simulink library "AttitudeControl"  (R2024a)
settings: Solver=VariableStepAuto  StartTime=0.0  StopTime=10.0  RelTol=1e-3
undefined symbols (not defined in the file): ATC_ANG_PIT_P, ATC_ANG_RLL_P, ATC_ANG_YAW_P, ATC_RAT_PIT_D, ATC_RAT_PIT_I, ATC_RAT_PIT_P, ATC_RAT_RLL_D, ATC_RAT_RLL_I, ATC_RAT_RLL_P, ATC_RAT_YAW_D, ATC_RAT_YAW_I, ATC_RAT_YAW_P
libraries: ArdupilotFunctions x3
settings Model: Creator=igmso  LastModifiedBy=igmso

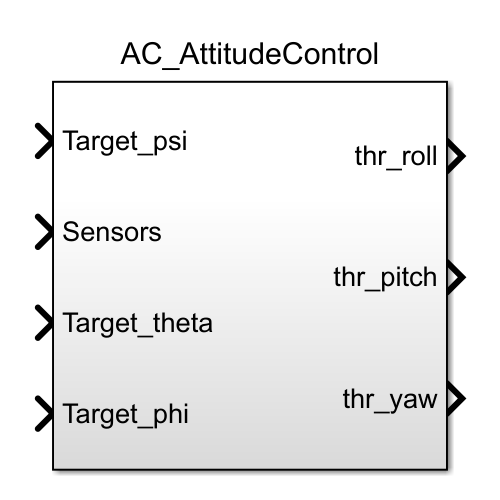
[thumbnail: Simulink's stored preview of the top-level diagram]
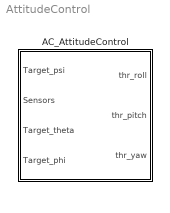
== system AttitudeControl ==
  AC_AttitudeControl : Subsystem

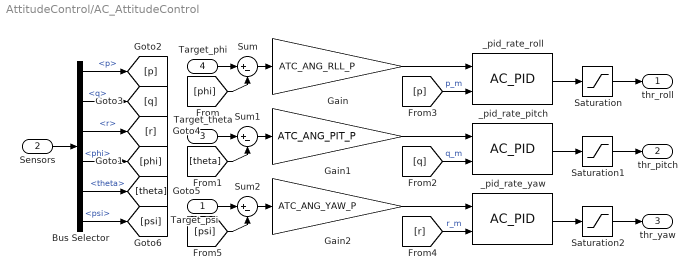
== system AttitudeControl/AC_AttitudeControl ==
  Target_psi : Inport
  Sensors : Inport  Port=2
  Target_theta : Inport  Port=3
  Target_phi : Inport  Port=4
  Bus Selector : BusSelector  OutputSignals=p,q,r,phi,theta,psi
  Gain : Gain  Gain=ATC_ANG_RLL_P
  Gain1 : Gain  Gain=ATC_ANG_PIT_P
  Gain2 : Gain  Gain=ATC_ANG_YAW_P
  Saturation : Saturate  UpperLimit=1  LowerLimit=-1
  Saturation1 : Saturate  UpperLimit=1  LowerLimit=-1
  Saturation2 : Saturate  UpperLimit=1  LowerLimit=-1
  Sum : Sum  Inputs=|+-
  Sum1 : Sum  Inputs=|+-
  Sum2 : Sum  Inputs=|+-
  _pid_rate_pitch : ArdupilotFunctions/AC_PID  P=ATC_RAT_PIT_P  I=ATC_RAT_PIT_I  D=ATC_RAT_PIT_D  FF=ATC_RAT_PIT_FF  D_FF=ATC_RAT_PIT_D_FF  FLTD=ATC_RAT_PIT_FLTD  FLTE=ATC_RAT_PIT_FLTE  FLTT=ATC_RAT_PIT_FLTT  IMAX=ATC_RAT_PIT_IMAX  ControlFreq=ATC_Freq
  _pid_rate_roll : ArdupilotFunctions/AC_PID  P=ATC_RAT_RLL_P  I=ATC_RAT_RLL_I  D=ATC_RAT_RLL_D  FF=ATC_RAT_RLL_FF  D_FF=ATC_RAT_RLL_D_FF  FLTD=ATC_RAT_RLL_FLTD  FLTE=ATC_RAT_RLL_FLTE  FLTT=ATC_RAT_RLL_FLTT  IMAX=ATC_RAT_RLL_IMAX  ControlFreq=ATC_Freq
  _pid_rate_yaw : ArdupilotFunctions/AC_PID  P=ATC_RAT_YAW_P  I=ATC_RAT_YAW_I  D=ATC_RAT_YAW_D  FF=ATC_RAT_YAW_FF  D_FF=ATC_RAT_YAW_D_FF  FLTD=ATC_RAT_YAW_FLTD  FLTE=ATC_RAT_YAW_FLTE  FLTT=ATC_RAT_YAW_FLTT  IMAX=ATC_RAT_YAW_IMAX  ControlFreq=ATC_Freq
  thr_roll : Outport
  thr_pitch : Outport  Port=2
  thr_yaw : Outport  Port=3
  wires:
  Saturation2/1 -> thr_yaw/1
  Saturation1/1 -> thr_pitch/1
  Saturation/1 -> thr_roll/1
  [psi] -> Sum2/2
  Target_psi/1 -> Sum2/1
  Sum2/1 -> Gain2/1
  Target_theta/1 -> Sum1/1
  [theta] -> Sum1/2
  Sum1/1 -> Gain1/1
  Gain/1 -> _pid_rate_roll/1
  Sum/1 -> Gain/1
  [phi] -> Sum/2
  Target_phi/1 -> Sum/1
  Bus Selector/6 -> [psi]  "<psi>"
  Bus Selector/5 -> [theta]  "<theta>"
  Bus Selector/4 -> [phi]  "<phi>"
  Gain1/1 -> _pid_rate_pitch/1
  _pid_rate_roll/1 -> Saturation/1
  Gain2/1 -> _pid_rate_yaw/1
  Bus Selector/3 -> [r]  "<r>"
  [r] -> _pid_rate_yaw/2  "r_m"
  _pid_rate_pitch/1 -> Saturation1/1
  Bus Selector/1 -> [p]  "<p>"
  [p] -> _pid_rate_roll/2  "p_m"
  Sensors/1 -> Bus Selector/1
  Bus Selector/2 -> [q]  "<q>"
  _pid_rate_yaw/1 -> Saturation2/1
  [q] -> _pid_rate_pitch/2  "q_m"
